simulink model "s_srv02_pos"  (Simulink 8.3)
settings: Solver=ode4  StartTime=0.0  StopTime=5  FixedStep=0.002  RelTol=1e-3  AbsTol=1e-6
undefined symbols (not defined in the file): K, K_AMP, ki, kp, kv, tau, VMAX_AMP, VMAX_DAC, wcf, zetaf
libraries: simulink_extras x2
settings Model: Creator=MLevis  LastModifiedBy=Student  ExtModeTrigDuration=10000  BufferReuse=off
settings SolverCC: PositivePriorityOrder=on
settings DataIOCC: LimitDataPoints=off
settings OptimizationCC: BlockReduction=off  BooleanDataType=off  OptimizeBlockIOStorage=off  BufferReuse=off  GlobalBufferReuse=off  ExpressionFolding=off  ExpressionDepthLimit=2147483647  LocalBlockOutputs=off  InitFltsAndDblsToZero=on
settings DebuggingCC: SaveWithParameterizedLinksMsg=none  SignalResolutionControl=TryResolveAllWithWarning  SolverPrmCheckMsg=none  MultiTaskDSMMsg=warning  MultiTaskCondExecSysMsg=none  FcnCallInpInsideContextMsg=UseLocalSettings
settings HardwareCC: TargetHWDeviceType=32-bit Generic
settings RTWCC: SystemTargetFile=quarc_windows.tlc  TemplateMakefile=quarc_default_tmf  Description=Quarc Win32 Target  ProcessScript=quarc_windows_make_rtw_hook  IncludeERTFirstTime=on
settings STFCustomTargetCC: TargetFcnLib=ansi_tfl_tmw.mat  TargetPreCompLibLocation=C:\PROGRA~2\QUARC\lib\2014a\windows\release  GeneratePreprocessorConditionals=Disable all  CPPClassGenCompliant=on  SystemTargetFile=quarc_windows.tlc
settings GRTTargetCC: TargetFcnLib=ansi_tfl_tmw.mat  TargetPreCompLibLocation=C:\PROGRA~2\QUARC\lib\2014a\windows\release  ParMdlRefBuildCompliant=off  CompOptLevelCompliant=off  ConcurrentExecutionCompliant=off  MatFileLogging=off  ExtMode=on  ExtModeMexFile=quarc_comm

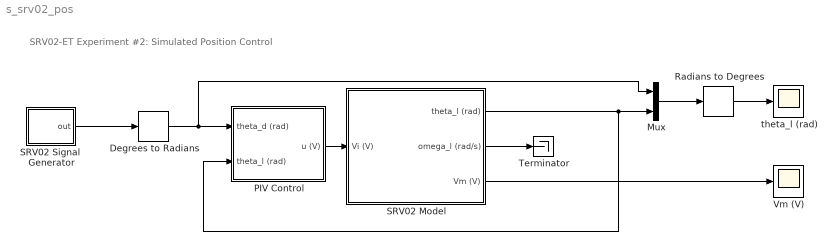
== system s_srv02_pos ==
  note: SRV02-ET Experiment #2: Simulated Position Control
  Degrees to Radians : simulink_extras/Transformations/Degrees to Radians
  Mux : Mux  Inputs=2
  PIV Control : Subsystem
  Radians to Degrees : simulink_extras/Transformations/Radians to Degrees
  SRV02 Model : Subsystem
  SRV02 Signal  Generator : Subsystem  mask(QET Signal Generator){sig_type=square, a=30, f=0.5}
      mask prompts: sig_type "Signal Type"; a "Amplitude"; f "Frequency (Hz)"
      mask help: Generates a square, triangular, or sinusoidal waveform of a specified amplitude and frequency.
      mask Help: Choose the type of signal to be generated from the drop-down "Signal Type" box. Enter the amplitude and the frequency desired for the signal. Note: frequency is in Hertz.
      mask TypeOptions sig_type: square | triangle | sine
      mask Display: plot([0 1 1 2 2 3 4 5 6], [-1 -1 1 1 -1 -1 1 -1 -1])
  Terminator : Terminator
  Vm (V) : Scope
      settings: TimeRange=5  YMin=-10  YMax=10  SaveName=data_vm
  theta_l (rad) : Scope
      settings: TimeRange=5  YMin=-1  YMax=1  SaveName=data_pos
  wires:
  SRV02 Model/2(omega_l (rad/s)) -> Terminator/1
  PIV Control/1(u (V)) -> SRV02 Model/1(Vi (V))
  SRV02 Model/1(theta_l (rad)) -> Mux/2, PIV Control/2(theta_l (rad))
  SRV02 Model/3(Vm (V)) -> Vm (V)/1
  Mux/1 -> Radians to Degrees/1
  SRV02 Signal  Generator/1(out) -> Degrees to Radians/1
  Degrees to Radians/1 -> PIV Control/1(theta_d (rad)), Mux/1
  Radians to Degrees/1 -> theta_l (rad)/1

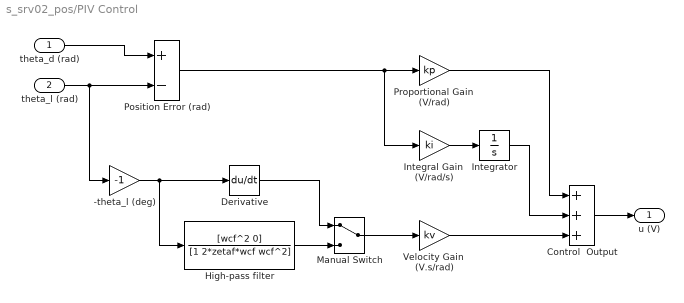
== system s_srv02_pos/PIV Control ==
  theta_d (rad) : Inport
  theta_l (rad) : Inport  Port=2
  -theta_l (deg) : Gain  Gain=-1
  Control  Output : Sum  Inputs=+++
  Derivative : Derivative
  High-pass filter : TransferFcn  Numerator=[wcf^2 0]  Denominator=[1 2*zetaf*wcf wcf^2]
  Integral Gain  (V/rad/s) : Gain  Gain=ki
  Integrator : Integrator
  Manual Switch : ManualSwitch
  Position Error (rad) : Sum  Inputs=+-
  Proportional Gain  (V/rad) : Gain  Gain=kp
  Velocity Gain  (V.s/rad) : Gain  Gain=kv
  u (V) : Outport
  wires:
  Proportional Gain  (V/rad)/1 -> Control  Output/1
  theta_d (rad)/1 -> Position Error (rad)/1
  Control  Output/1 -> u (V)/1
  theta_l (rad)/1 -> Position Error (rad)/2, -theta_l (deg)/1
  Position Error (rad)/1 -> Proportional Gain  (V/rad)/1, Integral Gain  (V/rad/s)/1
  -theta_l (deg)/1 -> Derivative/1, High-pass filter/1
  High-pass filter/1 -> Manual Switch/2
  Manual Switch/1 -> Velocity Gain  (V.s/rad)/1
  Derivative/1 -> Manual Switch/1
  Integral Gain  (V/rad/s)/1 -> Integrator/1
  Velocity Gain  (V.s/rad)/1 -> Control  Output/3
  Integrator/1 -> Control  Output/2

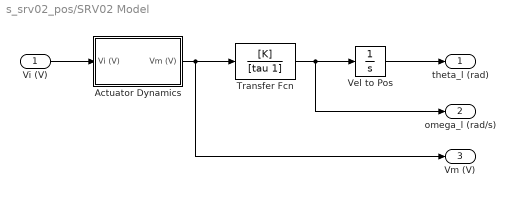
== system s_srv02_pos/SRV02 Model ==
  Vi (V) : Inport
  Actuator Dynamics : Subsystem
  Transfer Fcn : TransferFcn  Numerator=[K]  Denominator=[tau 1]
  Vel to Pos : Integrator
  theta_l (rad) : Outport
  omega_l (rad/s) : Outport  Port=2
  Vm (V) : Outport  Port=3
  wires:
  Transfer Fcn/1 -> omega_l (rad/s)/1, Vel to Pos/1
  Vel to Pos/1 -> theta_l (rad)/1
  Actuator Dynamics/1(Vm (V)) -> Transfer Fcn/1, Vm (V)/1
  Vi (V)/1 -> Actuator Dynamics/1(Vi (V))

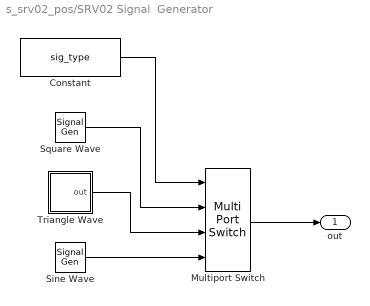
== system s_srv02_pos/SRV02 Signal  Generator ==
  Constant : Constant  Value=sig_type
  Multiport Switch : MultiPortSwitch
  Sine Wave : SignalGenerator  Amplitude=a  Frequency=f
  Square Wave : SignalGenerator  WaveForm=square  Amplitude=a  Frequency=f
  Triangle Wave : Subsystem
  out : Outport
  wires:
  Square Wave/1 -> Multiport Switch/2
  Triangle Wave/1(out) -> Multiport Switch/3
  Sine Wave/1 -> Multiport Switch/4
  Multiport Switch/1 -> out/1
  Constant/1 -> Multiport Switch/1

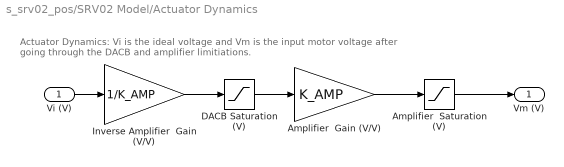
== system s_srv02_pos/SRV02 Model/Actuator Dynamics ==
  note: Actuator Dynamics: Vi is the ideal voltage and Vm is the
      | input motor voltage after going through the DACB and amplifier limitiations.
  Vi (V) : Inport
  Amplifier  Gain (V/V) : Gain  Gain=K_AMP
  Amplifier  Saturation (V) : Saturate  UpperLimit=VMAX_AMP  LowerLimit=-VMAX_AMP
  DACB Saturation (V) : Saturate  UpperLimit=VMAX_DAC  LowerLimit=-VMAX_DAC
  Inverse Amplifier  Gain (V/V) : Gain  Gain=1/K_AMP
  Vm (V) : Outport
  wires:
  Inverse Amplifier  Gain (V/V)/1 -> DACB Saturation (V)/1
  DACB Saturation (V)/1 -> Amplifier  Gain (V/V)/1
  Amplifier  Gain (V/V)/1 -> Amplifier  Saturation (V)/1
  Vi (V)/1 -> Inverse Amplifier  Gain (V/V)/1
  Amplifier  Saturation (V)/1 -> Vm (V)/1

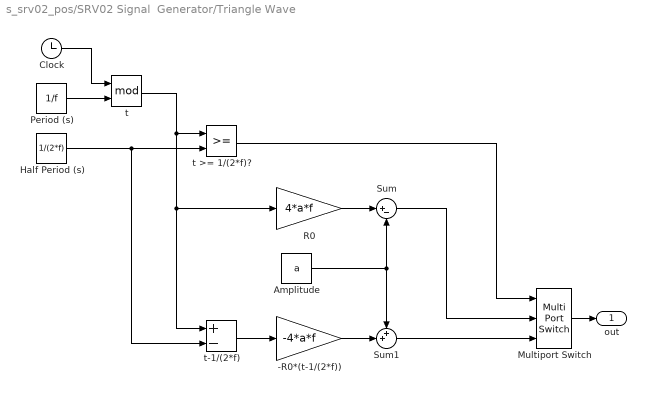
== system s_srv02_pos/SRV02 Signal  Generator/Triangle Wave ==
  -R0*(t-1/(2*f)) : Gain  Gain=-4*a*f
  Amplitude : Constant  Value=a
  Clock : Clock
  Half Period (s) : Constant  Value=1/(2*f)
  Multiport Switch : MultiPortSwitch  DataPortOrder=Zero-based contiguous  Inputs=2  zeroidx=on
  Period (s) : Constant  Value=1/f
  R0 : Gain  Gain=4*a*f
  Sum : Sum  Inputs=|+-
  Sum1 : Sum  Inputs=++|
  t : Math  Operator=mod  SaturateOnIntegerOverflow=on
  t >= 1/(2*f)? : RelationalOperator  OutDataTypeStr=boolean
  t-1/(2*f) : Sum  Inputs=+-
  out : Outport
  wires:
  Sum1/1 -> Multiport Switch/3
  Sum/1 -> Multiport Switch/2
  t >= 1/(2*f)?/1 -> Multiport Switch/1
  -R0*(t-1/(2*f))/1 -> Sum1/2
  Amplitude/1 -> Sum1/1, Sum/2
  R0/1 -> Sum/1
  t-1/(2*f)/1 -> -R0*(t-1/(2*f))/1
  Half Period (s)/1 -> t-1/(2*f)/2, t >= 1/(2*f)?/2
  t/1 -> t-1/(2*f)/1, R0/1, t >= 1/(2*f)?/1
  Period (s)/1 -> t/2
  Clock/1 -> t/1
  Multiport Switch/1 -> out/1
